simulink model "Monarch_DesignProblem_RevA_20210819_Samrudh_U_P"  (R2022a)
settings: Solver=VariableStepAuto  StartTime=0.0  StopTime=100  MinStep=0.001  RelTol=1e-3
undefined symbols (not defined in the file or in its folder): sigbuilder_block
libraries: simulink x4, slpidlib x2
settings Model: Creator=Corbin  LastModifiedBy=samrudh.untgodpr
settings SolverCC: InitialStep=0.001  AlgebraicLoopSolver=TrustRegion
settings DataIOCC: ReturnWorkspaceOutputs=off
settings DebuggingCC: UnconnectedInputMsg=warning  UnconnectedOutputMsg=warning  UnconnectedLineMsg=warning  SFMachineParentedDataDiag=warning  ArithmeticOperatorsInVariantConditions=warning
settings SFSimCC: SimUseLocalCustomCode=off  CustomCodeUndefinedFunction=UseInterfaceOnly
settings RTWCC: RTWUseLocalCustomCode=off

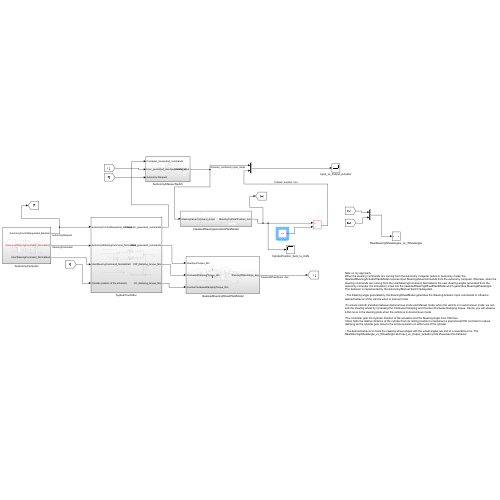
[thumbnail: Simulink's stored preview of the top-level diagram]
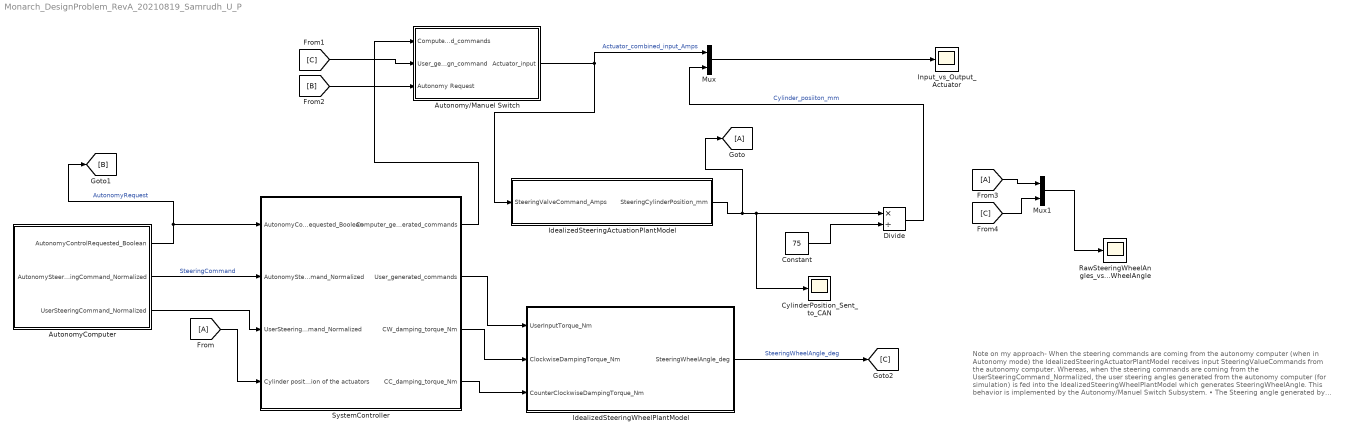
== system Monarch_DesignProblem_RevA_20210819_Samrudh_U_P ==
  note: Note on my approach-
      | When the steering commands are coming from the autonomy computer (when in Autonomy mode) the IdealizedSteeringActuatorPlantModel receives input SteeringValueCommands from the autonomy computer. Whereas, when the steering commands are coming from the UserSteeringCommand_Normalized, the user steering angles generated from the autonomy computer (for simulation) is fed into the IdealizedSteeringWheelPlantModel which generates SteeringWheelAngle. This behavior is implemented by the Autonomy/Manuel Switch Subsystem.
      |
      | • The Steering angle generated by the SteeringWheelModel generates the Steering Actuator input commands to influence desired behavior of the vehicle when in manuel mode.
      |
      | •To ensure smooth transition between Autonomous mode and Manuel mode, when the vehicle is in autonomous mode, we can lock the steering wheel by increasing the Clockwise Damping and Counter-Clockwise Damping torque. Hence, you will observe a flat curve in the steering plots when the vehicle is in Autonomous mode.
      |
      | •The controller gets the Cylinder Position of the actuators and the Steering Angle from CAN bus.
      | It then finds the relative distance of the cylinder from its resting position to implement a proportional PID controller to induce damping as the cylinder gets close to the lockout position on either end of the cylinder.
      |
      | • The desired behavior to track the steering wheel angles with the wheel angles are met at a resonable error. The RawSteeringWheelAngle_vs_WheelAngle and Input_vs_Output_Actuator plots showcase this behavior.
  Autonomy/Manuel Switch : Subsystem
  AutonomyComputer : Subsystem
  Constant : Constant  Value=75
  CylinderPosition_Sent_to_CAN : Scope
  Divide : Product  Inputs=*/
  From : From
  From3 : From
  Goto : Goto
  IdealizedSteeringActuationPlantModel : Subsystem
  IdealizedSteeringWheelPlantModel : Subsystem
  Input_vs_Output_Actuator : Scope
  Mux : Mux  Inputs=2
  Mux1 : Mux  Inputs=2
  RawSteeringWheelAngles_vs _WheelAngle : Scope
  SystemController : Subsystem
  wires:
  AutonomyComputer/1(AutonomyControlRequested_Boolean) -> [B], SystemController/1(AutonomyControlRequested_Boolean)  "AutonomyRequest"
  AutonomyComputer/2(AutonomySteeringCommand_Normalized) -> SystemController/2(AutonomySteeringCommand_Normalized)  "SteeringCommand"
  AutonomyComputer/3(UserSteeringCommand_Normalized) -> SystemController/3(UserSteeringCommand_Normalized)
  Constant/1 -> Divide/2
  SystemController/2(User_generated_commands) -> IdealizedSteeringWheelPlantModel/1(UserInputTorque_Nm)
  IdealizedSteeringActuationPlantModel/1(SteeringCylinderPosition_mm) -> Goto/1, Divide/1, CylinderPosition_Sent_to_CAN/1
  From/1 -> SystemController/4(Cylinder position of the actuators)
  SystemController/3(CW_damping_torque_Nm) -> IdealizedSteeringWheelPlantModel/2(ClockwiseDampingTorque_Nm)
  SystemController/4(CC_damping_torque_Nm) -> IdealizedSteeringWheelPlantModel/3(CounterClockwiseDampingTorque_Nm)
  SystemController/1(Computer_generated_commands) -> Autonomy/Manuel Switch/1(Computer_Generated_commands)
  Autonomy/Manuel Switch/1(Actuator_input) -> Mux/1, IdealizedSteeringActuationPlantModel/1(SteeringValveCommand_Amps)  "Actuator_combined_input_Amps"
  Mux/1 -> Input_vs_Output_Actuator/1
  [B] -> Autonomy/Manuel Switch/3("Autonomy Request ")
  [C] -> Autonomy/Manuel Switch/2(User_generated_steerign_command)
  IdealizedSteeringWheelPlantModel/1(SteeringWheelAngle_deg) -> [C]  "SteeringWheelAngle_deg"
  Divide/1 -> Mux/2  "Cylinder_posiiton_mm"
  From3/1 -> Mux1/1
  [C] -> Mux1/2
  Mux1/1 -> RawSteeringWheelAngles_vs _WheelAngle/1

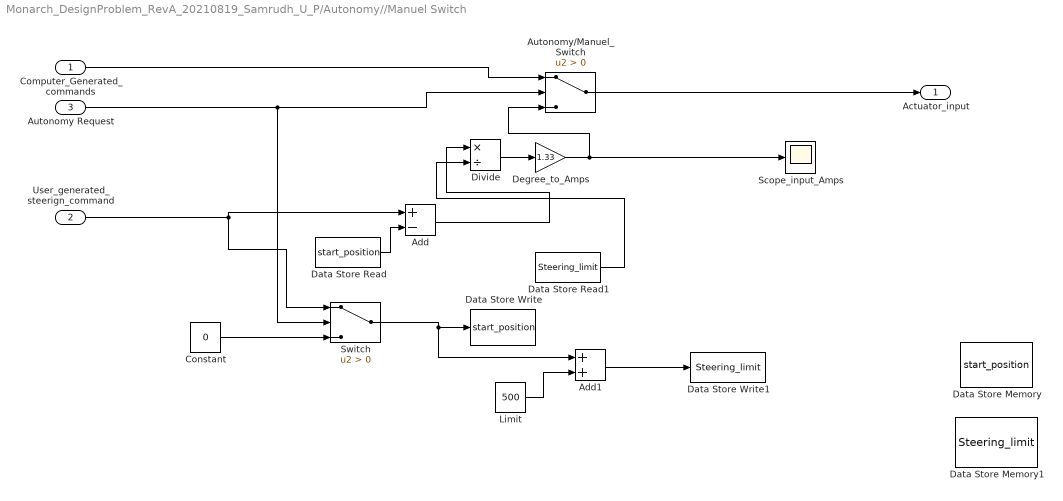
== system Monarch_DesignProblem_RevA_20210819_Samrudh_U_P/Autonomy//Manuel Switch ==
  Computer_Generated_commands : Inport
  User_generated_steerign_command : Inport  Port=2
  "Autonomy Request " : Inport  Port=3
  Add : Sum  Inputs=+-
  Add1 : Sum
  Autonomy/Manuel_Switch : Switch  Criteria=u2 > Threshold  SaturateOnIntegerOverflow=off  InputSameDT=off
  Constant : Constant  Value=0
  Data Store Memory : DataStoreMemory  DataStoreName=start_position  WriteAfterWriteMsg=warning  ShowAdditionalParam=off
  Data Store Memory1 : DataStoreMemory  DataStoreName=Steering_limit  WriteAfterWriteMsg=warning  ShowAdditionalParam=off
  Data Store Read : DataStoreRead  DataStoreName=start_position  IndexOptions=Index vector (dialog)  Indices=1  OutputSizes=1
  Data Store Read1 : DataStoreRead  DataStoreName=Steering_limit  IndexOptions=Index vector (dialog)  Indices=1  OutputSizes=1
  Data Store Write : DataStoreWrite  DataStoreName=start_position  IndexOptions=Index vector (dialog)  Indices=1  OutputSizes=1
  Data Store Write1 : DataStoreWrite  DataStoreName=Steering_limit  IndexOptions=Index vector (dialog)  Indices=1  OutputSizes=1
  Degree_to_Amps : Gain  Gain=1.33
  Divide : Product  Inputs=*/
  Limit : Constant  Value=500
  Scope_input_Amps : Scope
  Switch : Switch  Criteria=u2 > Threshold  SaturateOnIntegerOverflow=off  InputSameDT=off
  Actuator_input : Outport
  wires:
  Computer_Generated_commands/1 -> Autonomy/Manuel_Switch/1
  "Autonomy Request "/1 -> Switch/2, Autonomy/Manuel_Switch/2
  Autonomy/Manuel_Switch/1 -> Actuator_input/1
  User_generated_steerign_command/1 -> Add/1, Switch/1
  Constant/1 -> Switch/3
  Switch/1 -> Add1/1, Data Store Write/1
  Data Store Read/1 -> Add/2
  Add/1 -> Divide/1
  Add1/1 -> Data Store Write1/1
  Limit/1 -> Add1/2
  Data Store Read1/1 -> Divide/2
  Divide/1 -> Degree_to_Amps/1
  Degree_to_Amps/1 -> Autonomy/Manuel_Switch/3, Scope_input_Amps/1

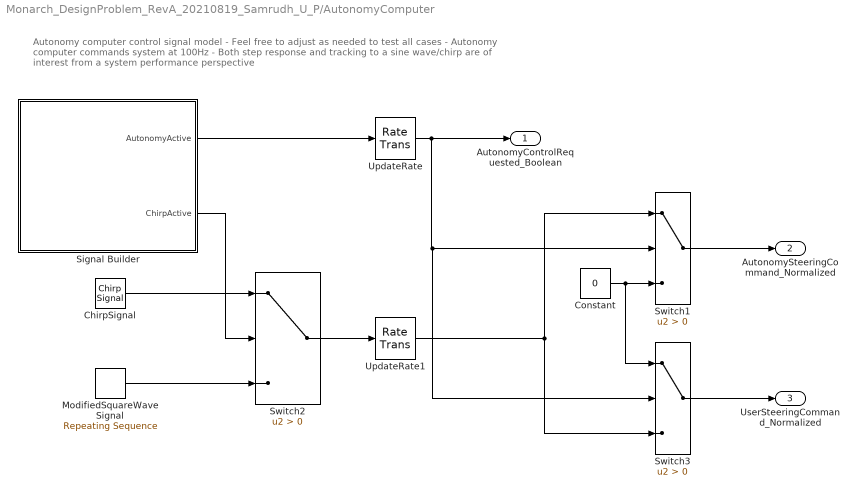
== system Monarch_DesignProblem_RevA_20210819_Samrudh_U_P/AutonomyComputer ==
  note: Autonomy computer control signal model
      | - Feel free to adjust as needed to test all cases
      | - Autonomy computer commands system at 100Hz
      | - Both step response and tracking to a sine wave/chirp are of interest from a system performance perspective
  ChirpSignal : simulink/Sources/Chirp Signal  f1=0.05  T=100  f2=0.5
  Constant : Constant  Value=0
  ModifiedSquareWaveSignal : simulink/Sources/Repeating Sequence  rep_seq_t=[0.000 1.000 1.100 3.000 3.100 5.000 5.100 6.000]  rep_seq_y=[0.000 0.000 1.000 1.000 -1.000 -1.000 0.000 0.000]
  Signal Builder : Subsystem  Tag=STV Subsys  LoadFcn=sigbuilder_block('load');  StartFcn=sigbuilder_block('start');  StopFcn=sigbuilder_block('stop');  ClipboardFcn=sigbuilder_block('clipboard');  mask(Sigbuilder block){tuvar=[0:10]}
      mask help: Simulink:masks:SigbuilderBlock_MD
      mask init:
      | if ~strcmp(get_param(bdroot(gcbh),'SimulationStatus'),'stopped') tuvar = sigbuilder_block('maskInit'); end
      settings: CopyFcn=sigbuilder_block('copy');  DeleteFcn=sigbuilder_block('delete');  ModelCloseFcn=sigbuilder_block('modelClose');  PreSaveFcn=sigbuilder_block('preSave');  PauseFcn=sigbuilder_block('pause');  ContinueFcn=sigbuilder_block('continue');  NameChangeFcn=sigbuilder_block('namechange');  OpenFcn=sigbuilder_block('open',[6 37.5 1428 548.25 ]);  CloseFcn=sigbuilder_block('close');
      mask Display: plot(0, 0, 100, 100,[2, 2, 32, 32, 2], [68, 8, 8, 68, 68],[32, 2], [38, 38], [32, 19, 2],[53, 60, 44], [32, 17, 17, 2],[16, 16, 31, 31]);txt = getActiveGroup(gcbh);text(2, 100, txt,'verticalAlignment', 'top');
  Switch1 : Switch  Criteria=u2 > Threshold  SaturateOnIntegerOverflow=off  InputSameDT=off
  Switch2 : Switch  Criteria=u2 > Threshold  SaturateOnIntegerOverflow=off  InputSameDT=off
  Switch3 : Switch  Criteria=u2 > Threshold  SaturateOnIntegerOverflow=off  InputSameDT=off
  UpdateRate : RateTransition  OutPortSampleTime=0.010
      settings: AttributesFormatString=%<OutPortSampleTime>
  UpdateRate1 : RateTransition  OutPortSampleTime=0.010
      settings: AttributesFormatString=%<OutPortSampleTime>
  AutonomyControlRequested_Boolean : Outport  VectorParamsAs1DForOutWhenUnconnected=off
  AutonomySteeringCommand_Normalized : Outport  Port=2  VectorParamsAs1DForOutWhenUnconnected=off
  UserSteeringCommand_Normalized : Outport  Port=3  VectorParamsAs1DForOutWhenUnconnected=off
  wires:
  ChirpSignal/1 -> Switch2/1
  ModifiedSquareWaveSignal/1 -> Switch2/3
  Switch2/1 -> UpdateRate1/1
  Signal Builder/1(AutonomyActive) -> UpdateRate/1
  Signal Builder/2(ChirpActive) -> Switch2/2
  UpdateRate/1 -> AutonomyControlRequested_Boolean/1, Switch3/2, Switch1/2
  UpdateRate1/1 -> Switch1/1, Switch3/3
  Switch1/1 -> AutonomySteeringCommand_Normalized/1
  Switch3/1 -> UserSteeringCommand_Normalized/1
  Constant/1 -> Switch3/1, Switch1/3

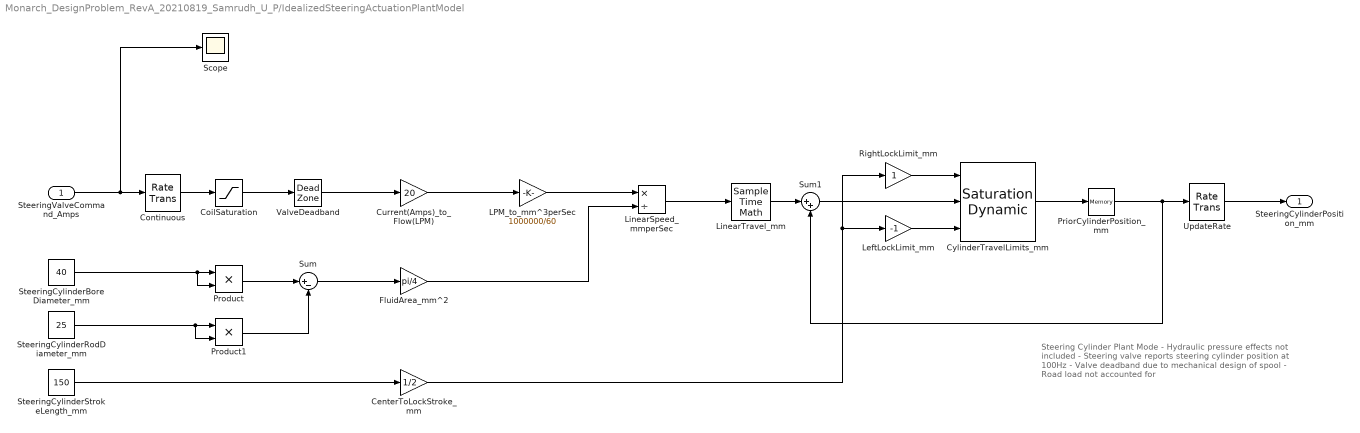
== system Monarch_DesignProblem_RevA_20210819_Samrudh_U_P/IdealizedSteeringActuationPlantModel ==
  note: Steering Cylinder Plant Mode
      | - Hydraulic pressure effects not included
      | - Steering valve reports steering cylinder position at 100Hz
      | - Valve deadband due to mechanical design of spool
      | - Road load not accounted for
  SteeringValveCommand_Amps : Inport
  CenterToLockStroke_mm : Gain  Gain=1/2
      settings: AttributesFormatString=%<Gain>
  CoilSaturation : Saturate  UpperLimit=1.33  LowerLimit=-1.33
      settings: AttributesFormatString=%<LowerLimit> to %<UpperLimit>
  Continuous : RateTransition  OutPortSampleTime=0
      settings: AttributesFormatString=%<OutPortSampleTime>
  Current(Amps)_to_Flow(LPM) : Gain  Gain=20
      settings: AttributesFormatString=%<Gain>
  CylinderTravelLimits_mm : simulink/Discontinuities/Saturation Dynamic  OutMin=[]  OutMax=[]  OutDataTypeStr=Inherit: Same as second input  OutDataType=fixdt(1, 16)  OutScaling=2^-10  DoSatur=off
  FluidArea_mm^2 : Gain  Gain=pi/4
      settings: AttributesFormatString=%<Gain>
  LPM_to_mm^3perSec : Gain  Gain=1000000/60
      settings: AttributesFormatString=%<Gain>
  LeftLockLimit_mm : Gain  Gain=-1
  LinearSpeed_mmperSec : Product  Inputs=*/
  LinearTravel_mm : SampleTimeMath  TsampMathOp=*
  PriorCylinderPosition_mm : Memory  InheritSampleTime=on
  Product : Product
  Product1 : Product
  RightLockLimit_mm : Gain
  Scope : Scope
  SteeringCylinderBoreDiameter_mm : Constant  Value=40
  SteeringCylinderRodDiameter_mm : Constant  Value=25
  SteeringCylinderStrokeLength_mm : Constant  Value=150
  Sum : Sum  Inputs=|+-
  Sum1 : Sum  Inputs=|++
  UpdateRate : RateTransition  OutPortSampleTime=0.010
      settings: AttributesFormatString=%<OutPortSampleTime>
  ValveDeadband : DeadZone  LowerValue=-0.33  UpperValue=0.33
      settings: AttributesFormatString=%<LowerValue> to %<UpperValue>
  SteeringCylinderPosition_mm : Outport  VectorParamsAs1DForOutWhenUnconnected=off
  wires:
  SteeringValveCommand_Amps/1 -> Scope/1, Continuous/1
  CoilSaturation/1 -> ValveDeadband/1
  ValveDeadband/1 -> Current(Amps)_to_Flow(LPM)/1
  Current(Amps)_to_Flow(LPM)/1 -> LPM_to_mm^3perSec/1
  SteeringCylinderBoreDiameter_mm/1 -> Product/2, Product/1
  SteeringCylinderRodDiameter_mm/1 -> Product1/2, Product1/1
  Product/1 -> Sum/1
  Product1/1 -> Sum/2
  Sum/1 -> FluidArea_mm^2/1
  SteeringCylinderStrokeLength_mm/1 -> CenterToLockStroke_mm/1
  LPM_to_mm^3perSec/1 -> LinearSpeed_mmperSec/1
  FluidArea_mm^2/1 -> LinearSpeed_mmperSec/2
  LinearSpeed_mmperSec/1 -> LinearTravel_mm/1
  CenterToLockStroke_mm/1 -> LeftLockLimit_mm/1, RightLockLimit_mm/1
  RightLockLimit_mm/1 -> CylinderTravelLimits_mm/1
  LeftLockLimit_mm/1 -> CylinderTravelLimits_mm/3
  LinearTravel_mm/1 -> Sum1/1
  Sum1/1 -> CylinderTravelLimits_mm/2
  PriorCylinderPosition_mm/1 -> Sum1/2, UpdateRate/1
  CylinderTravelLimits_mm/1 -> PriorCylinderPosition_mm/1
  UpdateRate/1 -> SteeringCylinderPosition_mm/1
  Continuous/1 -> CoilSaturation/1

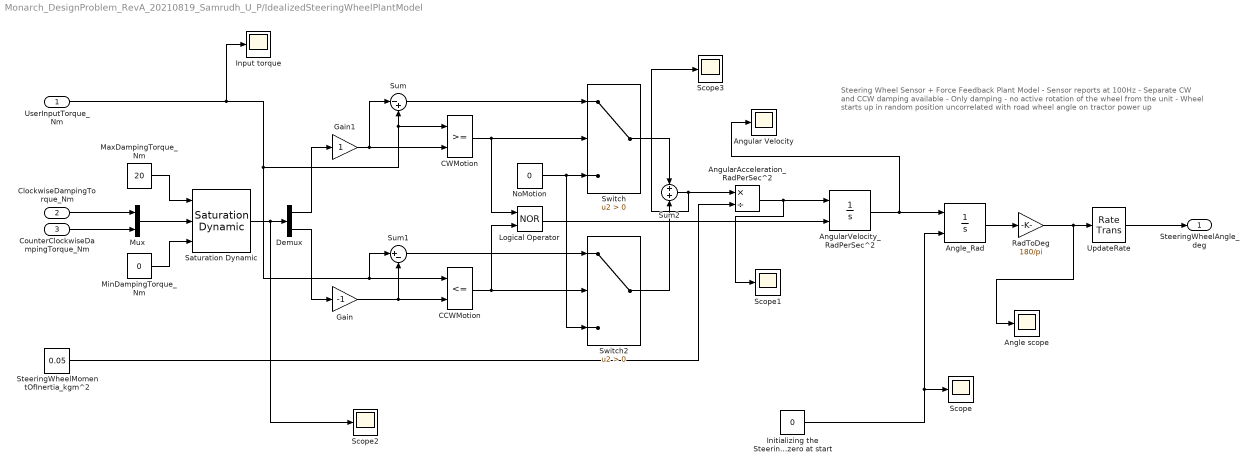
== system Monarch_DesignProblem_RevA_20210819_Samrudh_U_P/IdealizedSteeringWheelPlantModel ==
  note: Steering Wheel Sensor + Force Feedback Plant Model
      | - Sensor reports at 100Hz
      | - Separate CW and CCW damping available
      | - Only damping - no active rotation of the wheel from the unit
      | - Wheel starts up in random position uncorrelated with road wheel angle on tractor power up
  UserInputTorque_Nm : Inport
  ClockwiseDampingTorque_Nm : Inport  Port=2
  CounterClockwiseDampingTorque_Nm : Inport  Port=3
  Angle scope : Scope
  Angle_Rad : Integrator  InitialConditionSource=external
  Angular Velocity : Scope
  AngularAcceleration_RadPerSec^2 : Product  Inputs=*/
  AngularVelocity_RadPerSec^2 : Integrator  ExternalReset=level
  CCWMotion : RelationalOperator  Operator=<=  OutDataTypeStr=boolean  RndMeth=Simplest  InputSameDT=off
  CWMotion : RelationalOperator  OutDataTypeStr=boolean  RndMeth=Simplest  InputSameDT=off
  Demux : Demux  Outputs=2
  Gain : Gain  Gain=-1
  Gain1 : Gain
  Initializing the Steering wheel psition to zero at start : Constant  Value=0
  Input torque : Scope
  Logical Operator : Logic  Operator=NOR  AllPortsSameDT=off  OutDataTypeStr=boolean
  MaxDampingTorque_Nm : Constant  Value=20
  MinDampingTorque_Nm : Constant  Value=0
  Mux : Mux  Inputs=2
  NoMotion : Constant  Value=0
  RadToDeg : Gain  Gain=180/pi
      settings: AttributesFormatString=%<Gain>
  Saturation Dynamic : simulink/Discontinuities/Saturation Dynamic  OutMin=[]  OutMax=[]  OutDataTypeStr=Inherit: Same as second input  OutDataType=fixdt(1, 16)  OutScaling=2^-10  DoSatur=off
  Scope{,1..3} (4 alike) : Scope
  SteeringWheelMomentOfInertia_kgm^2 : Constant  Value=0.05
  Sum : Sum  Inputs=|-+
  Sum1 : Sum  Inputs=|+-
  Sum2 : Sum  Inputs=+|+
  Switch : Switch  Criteria=u2 > Threshold  SaturateOnIntegerOverflow=off  InputSameDT=off
  Switch2 : Switch  Criteria=u2 > Threshold  SaturateOnIntegerOverflow=off  InputSameDT=off
  UpdateRate : RateTransition  OutPortSampleTime=0.010
      settings: AttributesFormatString=%<OutPortSampleTime>
  SteeringWheelAngle_deg : Outport  VectorParamsAs1DForOutWhenUnconnected=off
  wires:
  UserInputTorque_Nm/1 -> Input torque/1, Sum1/1, CCWMotion/1, CWMotion/1, Sum/2
  ClockwiseDampingTorque_Nm/1 -> Mux/1
  Sum/1 -> Switch/1
  CWMotion/1 -> Logical Operator/1, Switch/2
  CounterClockwiseDampingTorque_Nm/1 -> Mux/2
  Gain/1 -> CCWMotion/2, Sum1/2
  NoMotion/1 -> Switch2/3, Switch/3
  CCWMotion/1 -> Logical Operator/2, Switch2/2
  Mux/1 -> Saturation Dynamic/2
  MaxDampingTorque_Nm/1 -> Saturation Dynamic/1
  MinDampingTorque_Nm/1 -> Saturation Dynamic/3
  Saturation Dynamic/1 -> Scope2/1, Demux/1
  Demux/1 -> Gain1/1
  Demux/2 -> Gain/1
  Sum1/1 -> Switch2/1
  Gain1/1 -> Sum/1, CWMotion/2
  Switch/1 -> Sum2/1
  Switch2/1 -> Sum2/2
  Sum2/1 -> AngularAcceleration_RadPerSec^2/1, Scope3/1
  SteeringWheelMomentOfInertia_kgm^2/1 -> AngularAcceleration_RadPerSec^2/2
  AngularAcceleration_RadPerSec^2/1 -> Scope1/1, AngularVelocity_RadPerSec^2/1
  AngularVelocity_RadPerSec^2/1 -> Angular Velocity/1, Angle_Rad/1
  Angle_Rad/1 -> RadToDeg/1
  RadToDeg/1 -> Angle scope/1, UpdateRate/1
  Logical Operator/1 -> AngularVelocity_RadPerSec^2/2
  UpdateRate/1 -> SteeringWheelAngle_deg/1
  Initializing the Steering wheel psition to zero at start/1 -> Scope/1, Angle_Rad/2

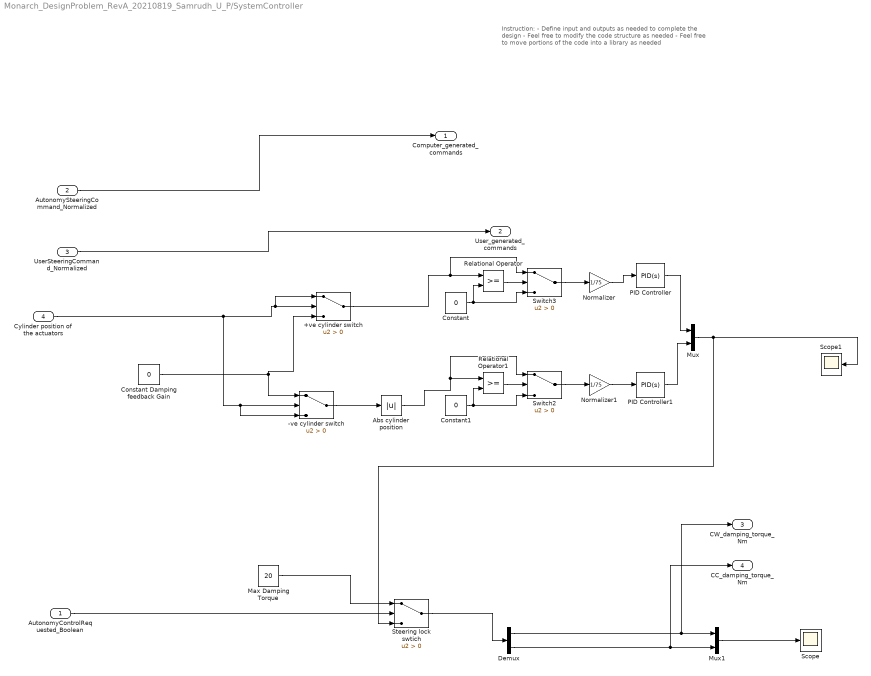
== system Monarch_DesignProblem_RevA_20210819_Samrudh_U_P/SystemController ==
  note: Instruction:
      | - Define input and outputs as needed to complete the design
      | - Feel free to modify the code structure as needed
      | - Feel free to move portions of the code into a library as needed
  AutonomyControlRequested_Boolean : Inport
  AutonomySteeringCommand_Normalized : Inport  Port=2
  UserSteeringCommand_Normalized : Inport  Port=3
  Cylinder position of the actuators : Inport  Port=4
  +ve cylinder switch : Switch  Criteria=u2 > Threshold  SaturateOnIntegerOverflow=off  InputSameDT=off
  -ve cylinder switch : Switch  Criteria=u2 > Threshold  SaturateOnIntegerOverflow=off  InputSameDT=off
  Abs cylinder position : Abs  SaturateOnIntegerOverflow=off
  Constant : Constant  Value=0
  Constant Damping feedback Gain : Constant  Value=0
  Constant1 : Constant  Value=0
  Demux : Demux  Outputs=2
  Max Damping Torque : Constant  Value=20
  Mux : Mux  Inputs=2
  Mux1 : Mux  Inputs=2
  Normalizer : Gain  Gain=1/75
  Normalizer1 : Gain  Gain=1/75
  PID Controller : slpidlib/PID Controller  Controller=PID  Form=Parallel  TimeDomain=Continuous-time  UseExternalTs=off  SampleTime=-1  IntegratorMethod=Forward Euler  FilterMethod=Forward Euler  ControllerParametersSource=internal  P=1.4  I=0  UseKiTs=off  D=0  N=100  UseFilter=on  TunerSelectOption=Transfer Function Based (PID Tuner App)  InitialConditionSource=internal  InitialConditionForIntegrator=0  InitialConditionForFilter=0  DifferentiatorICPrevScaledInput=0  ExternalReset=none  TrackingMode=off  Kt=1  LimitOutput=off  SatLimitsSource=internal  UpperSaturationLimit=inf  LowerSaturationLimit=-inf  LinearizeAsGain=on  AntiWindupMode=none  Kb=1  POutMin=[]  POutMax=[]  IOutMin=[]  IOutMax=[]  DOutMin=[]  DOutMax=[]  NOutMin=[]  NOutMax=[]  SumOutMin=[]  SumOutMax=[]  SaturationOutMin=[]  SaturationOutMax=[]  PParamMin=[]  PParamMax=[]  IParamMin=[]  IParamMax=[]  DParamMin=[]  DParamMax=[]  NParamMin=[]  NParamMax=[]  KbParamMin=[]  KbParamMax=[]  KtParamMin=[]  KtParamMax=[]  KbOutMin=[]  KbOutMax=[]  KtOutMin=[]  KtOutMax=[]  IntegratorOutMin=[]  IntegratorOutMax=[]  FilterOutMin=[]  FilterOutMax=[]  SumI1OutMin=[]  SumI1OutMax=[]  SumI2OutMin=[]  SumI2OutMax=[]  SumI3OutMin=[]  SumI3OutMax=[]  SumI4OutMin=[]  SumI4OutMax=[]  SumDOutMin=[]  SumDOutMax=[]  DifferentiatorOutMin=[]  DifferentiatorOutMax=[]  FilterDiffOutCoefMin=[]  FilterDiffOutCoefMax=[]  ReciprocalOutMin=[]  ReciprocalOutMax=[]  SumDenOutMin=[]  SumDenOutMax=[]  SumNumOutMin=[]  SumNumOutMax=[]  DivideOutMin=[]  DivideOutMax=[]  UdiffTsProdOutMin=[]  UdiffTsProdOutMax=[]  NTsProdOutMin=[]  NTsProdOutMax=[]  UintegralTsProdOutMin=[]  UintegralTsProdOutMax=[]  UngainTsProdOutMin=[]  UngainTsProdOutMax=[]  IntegratorContinuousStateAttributes=''  IntegratorStateMustResolveToSignalObject=off  IntegratorRTWStateStorageClass=Auto  FilterContinuousStateAttributes=''  FilterStateMustResolveToSignalObject=off  FilterRTWStateStorageClass=Auto  ParallelPVariant=InternalParameters  IdealPVariant=Disabled  IVariant=InternalParameters  DVariant=InternalParameters  IntegratorVariant=Continuous  SatVariant=Disabled  AWVariant=Passthrough  PCopyVariant=Disabled  TRVariant=Disabled  FdbkBlocksVariant=Forward  IdealPFdbkVariant=Disabled  SatFdbkVariant=Disabled  DerivativeFilterVariant=ContFilter  NVariant=InternalParameters  NCopyVariant=Disabled  FilterICVariant=InternalICsFilter  IntegratorICVariant=InternalICs  ExternalResetVariant=Disabled  TRSumVariant=Passthrough  SumFdbkVariant=Disabled  SumVariant=Sum_PID  TsampFilterVariant=InternalTs  TsampNgainVariant=Passthrough  TsampIntegralVariant=Passthrough  ExternalSaturationOutDataTypeStr=Inherit: Same as second input  aMode=0
  PID Controller1 : slpidlib/PID Controller  Controller=PID  Form=Parallel  TimeDomain=Continuous-time  UseExternalTs=off  SampleTime=-1  IntegratorMethod=Forward Euler  FilterMethod=Forward Euler  ControllerParametersSource=internal  P=1.4  I=0  UseKiTs=off  D=0  N=100  UseFilter=on  TunerSelectOption=Transfer Function Based (PID Tuner App)  InitialConditionSource=internal  InitialConditionForIntegrator=0  InitialConditionForFilter=0  DifferentiatorICPrevScaledInput=0  ExternalReset=none  TrackingMode=off  Kt=1  LimitOutput=off  SatLimitsSource=internal  UpperSaturationLimit=inf  LowerSaturationLimit=-inf  LinearizeAsGain=on  AntiWindupMode=none  Kb=1  POutMin=[]  POutMax=[]  IOutMin=[]  IOutMax=[]  DOutMin=[]  DOutMax=[]  NOutMin=[]  NOutMax=[]  SumOutMin=[]  SumOutMax=[]  SaturationOutMin=[]  SaturationOutMax=[]  PParamMin=[]  PParamMax=[]  IParamMin=[]  IParamMax=[]  DParamMin=[]  DParamMax=[]  NParamMin=[]  NParamMax=[]  KbParamMin=[]  KbParamMax=[]  KtParamMin=[]  KtParamMax=[]  KbOutMin=[]  KbOutMax=[]  KtOutMin=[]  KtOutMax=[]  IntegratorOutMin=[]  IntegratorOutMax=[]  FilterOutMin=[]  FilterOutMax=[]  SumI1OutMin=[]  SumI1OutMax=[]  SumI2OutMin=[]  SumI2OutMax=[]  SumI3OutMin=[]  SumI3OutMax=[]  SumI4OutMin=[]  SumI4OutMax=[]  SumDOutMin=[]  SumDOutMax=[]  DifferentiatorOutMin=[]  DifferentiatorOutMax=[]  FilterDiffOutCoefMin=[]  FilterDiffOutCoefMax=[]  ReciprocalOutMin=[]  ReciprocalOutMax=[]  SumDenOutMin=[]  SumDenOutMax=[]  SumNumOutMin=[]  SumNumOutMax=[]  DivideOutMin=[]  DivideOutMax=[]  UdiffTsProdOutMin=[]  UdiffTsProdOutMax=[]  NTsProdOutMin=[]  NTsProdOutMax=[]  UintegralTsProdOutMin=[]  UintegralTsProdOutMax=[]  UngainTsProdOutMin=[]  UngainTsProdOutMax=[]  IntegratorContinuousStateAttributes=''  IntegratorStateMustResolveToSignalObject=off  IntegratorRTWStateStorageClass=Auto  FilterContinuousStateAttributes=''  FilterStateMustResolveToSignalObject=off  FilterRTWStateStorageClass=Auto  ParallelPVariant=InternalParameters  IdealPVariant=Disabled  IVariant=InternalParameters  DVariant=InternalParameters  IntegratorVariant=Continuous  SatVariant=Disabled  AWVariant=Passthrough  PCopyVariant=Disabled  TRVariant=Disabled  FdbkBlocksVariant=Forward  IdealPFdbkVariant=Disabled  SatFdbkVariant=Disabled  DerivativeFilterVariant=ContFilter  NVariant=InternalParameters  NCopyVariant=Disabled  FilterICVariant=InternalICsFilter  IntegratorICVariant=InternalICs  ExternalResetVariant=Disabled  TRSumVariant=Passthrough  SumFdbkVariant=Disabled  SumVariant=Sum_PID  TsampFilterVariant=InternalTs  TsampNgainVariant=Passthrough  TsampIntegralVariant=Passthrough  ExternalSaturationOutDataTypeStr=Inherit: Same as second input  aMode=0
  Relational Operator : RelationalOperator  OutDataTypeStr=boolean  RndMeth=Simplest  InputSameDT=off
  Relational Operator1 : RelationalOperator  OutDataTypeStr=boolean  RndMeth=Simplest  InputSameDT=off
  Scope : Scope
  Scope1 : Scope
  Steering lock swtich : Switch  Criteria=u2 > Threshold  SaturateOnIntegerOverflow=off  InputSameDT=off
  Switch2 : Switch  Criteria=u2 > Threshold  SaturateOnIntegerOverflow=off  InputSameDT=off
  Switch3 : Switch  Criteria=u2 > Threshold  SaturateOnIntegerOverflow=off  InputSameDT=off
  Computer_generated_commands : Outport  VectorParamsAs1DForOutWhenUnconnected=off
  User_generated_commands : Outport  Port=2  VectorParamsAs1DForOutWhenUnconnected=off
  CW_damping_torque_Nm : Outport  Port=3
  CC_damping_torque_Nm : Outport  Port=4
  wires:
  AutonomyControlRequested_Boolean/1 -> Steering lock swtich/2
  Cylinder position of the actuators/1 -> +ve cylinder switch/2, +ve cylinder switch/1, -ve cylinder switch/2, -ve cylinder switch/3
  Constant Damping feedback Gain/1 -> -ve cylinder switch/1, +ve cylinder switch/3
  Max Damping Torque/1 -> Steering lock swtich/1
  Demux/1 -> CW_damping_torque_Nm/1, Mux1/1
  Demux/2 -> CC_damping_torque_Nm/1, Mux1/2
  Mux1/1 -> Scope/1
  AutonomySteeringCommand_Normalized/1 -> Computer_generated_commands/1
  UserSteeringCommand_Normalized/1 -> User_generated_commands/1
  Steering lock swtich/1 -> Demux/1
  Constant/1 -> Relational Operator/2, Switch3/3
  +ve cylinder switch/1 -> Switch3/1, Relational Operator/1
  Relational Operator/1 -> Switch3/2
  Switch3/1 -> Normalizer/1
  PID Controller/1 -> Mux/1
  Switch2/1 -> Normalizer1/1
  Relational Operator1/1 -> Switch2/2
  -ve cylinder switch/1 -> Abs cylinder position/1
  Constant1/1 -> Relational Operator1/2, Switch2/3
  Abs cylinder position/1 -> Switch2/1, Relational Operator1/1
  PID Controller1/1 -> Mux/2
  Normalizer/1 -> PID Controller/1
  Normalizer1/1 -> PID Controller1/1
  Mux/1 -> Steering lock swtich/3, Scope1/1

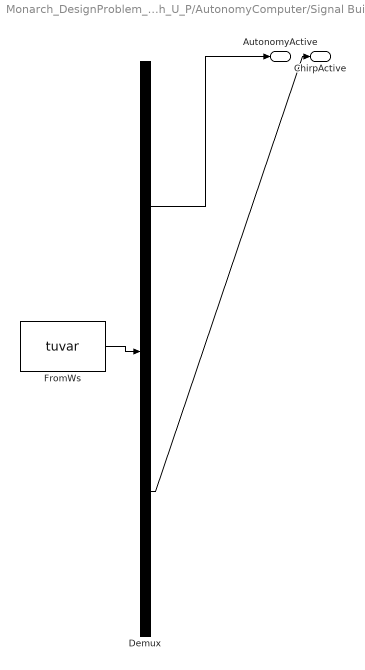
== system Monarch_DesignProblem_RevA_20210819_Samrudh_U_P/AutonomyComputer/Signal Builder ==
  Demux : Demux  Tag=STV Demux  Outputs=2
      settings: DisplayOption=none
  FromWs : FromWorkspace  Tag=STV FromWs  VariableName=tuvar
      SigBuilderData=|
      | common.afterFinalStr = 'Extrapolate'
      | common.sampleTime = 0
      | dataSet.timeRange = [0 100]
      | dataSet.name = 'Group 1'
      | sbobj.Groups.Name = 'Group 1'
      | sbobj.Groups.Signals(1).Name = 'AutonomyActive'
      | sbobj.Groups.Signals(1).XData = [0 8 8 52 52 70 70 90 90 100]
      | sbobj.Groups.Signals(1).YData = [0 0 1 1 0 0 1 1 0 0]
      | sbobj.Groups.Signals(2).Name = 'ChirpActive'
      | sbobj.Groups.Signals(2).XData = [0 10 10 30 30 60 60 80 80 100]
      | sbobj.Groups.Signals(2).YData = [0 0 1 1 0 0 1 1 0 0]
      | sbobj.Groups.TimeRange = [0 100]
  AutonomyActive : Outport  Tag=STV Outport  VectorParamsAs1DForOutWhenUnconnected=off
  ChirpActive : Outport  Tag=STV Outport  Port=2  VectorParamsAs1DForOutWhenUnconnected=off
  wires:
  Demux/1 -> AutonomyActive/1
  FromWs/1 -> Demux/1
  Demux/2 -> ChirpActive/1
